simulink model "Correcteur_rst"  (R2022b)
settings: Solver=VariableStepAuto  StartTime=0.0  StopTime=10.0  RelTol=1e-3
undefined symbols (not defined in the file): M, numR, numS, numT, Te
settings Model: Creator=antoi  LastModifiedBy=antoi

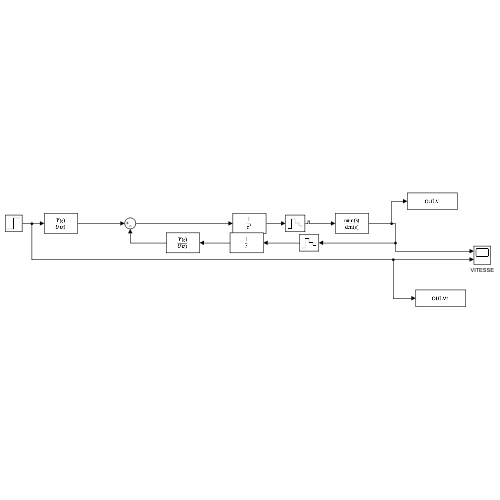
[thumbnail: Simulink's stored preview of the top-level diagram]
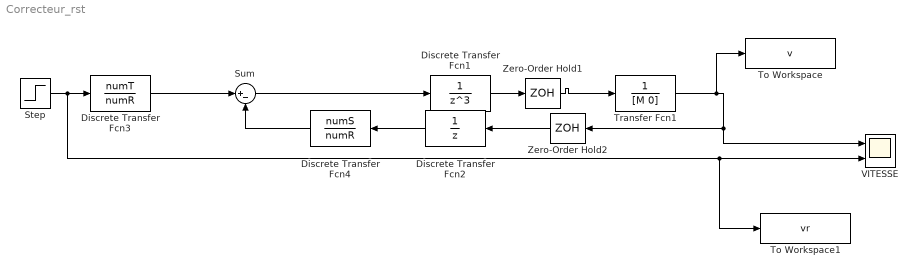
== system Correcteur_rst ==
  Discrete Transfer Fcn1 : DiscreteTransferFcn  Numerator=1  Denominator=[1 0 0 0]  SampleTime=Te
  Discrete Transfer Fcn2 : DiscreteTransferFcn  Numerator=1  Denominator=[1 0]  SampleTime=Te
  Discrete Transfer Fcn3 : DiscreteTransferFcn  Numerator=numT  Denominator=numR  SampleTime=Te
  Discrete Transfer Fcn4 : DiscreteTransferFcn  Numerator=numS  Denominator=numR  SampleTime=Te
  Step : Step  Time=0  SampleTime=0
  Sum : Sum  Inputs=|+-
  To Workspace : ToWorkspace  VariableName=v  SaveFormat=Timeseries  SampleTime=-1
  To Workspace1 : ToWorkspace  VariableName=vr  SaveFormat=Timeseries  SampleTime=-1
  Transfer Fcn1 : TransferFcn  Denominator=[M 0]
  VITESSE : Scope  NumInputPorts=2
  Zero-Order Hold1 : ZeroOrderHold  SampleTime=Te
  Zero-Order Hold2 : ZeroOrderHold  SampleTime=Te
  wires:
  Discrete Transfer Fcn2/1 -> Discrete Transfer Fcn4/1
  Zero-Order Hold1/1 -> Transfer Fcn1/1
  Discrete Transfer Fcn3/1 -> Sum/1
  Zero-Order Hold2/1 -> Discrete Transfer Fcn2/1
  Sum/1 -> Discrete Transfer Fcn1/1
  Transfer Fcn1/1 -> To Workspace/1, VITESSE/1, Zero-Order Hold2/1
  Discrete Transfer Fcn1/1 -> Zero-Order Hold1/1
  Discrete Transfer Fcn4/1 -> Sum/2
  Step/1 -> To Workspace1/1, VITESSE/2, Discrete Transfer Fcn3/1
